simulink model "DK_Quydao_Control_PID1"  (R2020b)
settings: Solver=VariableStepAuto  StartTime=0.0  StopTime=20  RelTol=1e-3
undefined symbols (not defined in the file or in its folder): Kd1, Kd2, Ki1, Ki2, Kp1, Kp2
settings Model: Creator=ADMIN  LastModifiedBy=Admin
settings DataIOCC: ReturnWorkspaceOutputs=off
settings DebuggingCC: ArithmeticOperatorsInVariantConditions=warning
settings SFSimCC: CustomCodeUndefinedFunction=UseInterfaceOnly

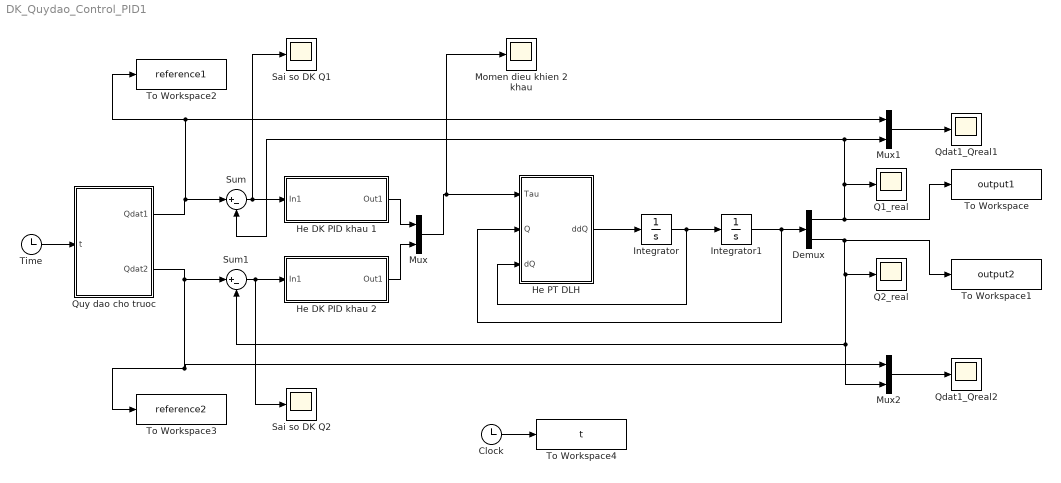
== system DK_Quydao_Control_PID1 ==
  Clock : Clock
  Demux : Demux  Outputs=2
  He DK PID khau 1 : Subsystem
  He DK PID khau 2 : Subsystem
  He PT DLH : MATLAB Function  TreatAsAtomicUnit=on
  Integrator : Integrator
  Integrator1 : Integrator  InitialCondition=[0;2]
  Momen dieu khien 2 khau : Scope
  Mux : Mux  Inputs=2
  Mux1 : Mux  Inputs=2
  Mux2 : Mux  Inputs=2
  Q1_real : Scope
  Q2_real : Scope
  Qdat1_Qreal1 : Scope
  Qdat1_Qreal2 : Scope
  Quy dao cho truoc : MATLAB Function  TreatAsAtomicUnit=on
  Sai so DK Q1 : Scope
  Sai so DK Q2 : Scope
  Sum : Sum  Inputs=|+-
  Sum1 : Sum  Inputs=|+-
  Time : Clock
  To Workspace : ToWorkspace  VariableName=output1  SampleTime=-1
  To Workspace1 : ToWorkspace  VariableName=output2  SampleTime=-1
  To Workspace2 : ToWorkspace  VariableName=reference1  SampleTime=-1
  To Workspace3 : ToWorkspace  VariableName=reference2  SampleTime=-1
  To Workspace4 : ToWorkspace  VariableName=t  SampleTime=-1
  wires:
  He PT DLH/1(ddQ) -> Integrator/1
  Mux/1 -> Momen dieu khien 2 khau/1, He PT DLH/1(Tau)
  He DK PID khau 1/1(Out1) -> Mux/1
  He DK PID khau 2/1(Out1) -> Mux/2
  Sum/1 -> Sai so DK Q1/1, He DK PID khau 1/1(In1)
  Quy dao cho truoc/1(Qdat1) -> Mux1/1, To Workspace2/1, Sum/1
  Sum1/1 -> Sai so DK Q2/1, He DK PID khau 2/1(In1)
  Quy dao cho truoc/2(Qdat2) -> Sum1/1, To Workspace3/1, Mux2/1
  Mux2/1 -> Qdat1_Qreal2/1
  Mux1/1 -> Qdat1_Qreal1/1
  Integrator1/1 -> He PT DLH/2(Q), Demux/1
  Integrator/1 -> He PT DLH/3(dQ), Integrator1/1
  Demux/1 -> To Workspace/1, Sum/2, Mux1/2, Q1_real/1
  Demux/2 -> To Workspace1/1, Sum1/2, Mux2/2, Q2_real/1
  Time/1 -> Quy dao cho truoc/1(t)
  Clock/1 -> To Workspace4/1

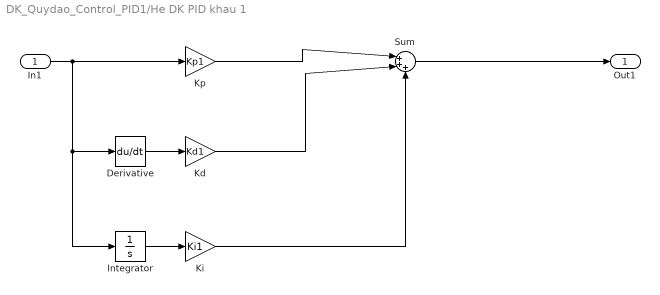
== system DK_Quydao_Control_PID1/He DK PID khau 1 ==
  In1 : Inport
  Derivative : Derivative
  Integrator : Integrator
  Kd : Gain  Gain=Kd1
  Ki : Gain  Gain=Ki1
  Kp : Gain  Gain=Kp1
  Sum : Sum  Inputs=|+++
  Out1 : Outport  VectorParamsAs1DForOutWhenUnconnected=off
  wires:
  In1/1 -> Derivative/1, Integrator/1, Kp/1
  Kp/1 -> Sum/1
  Integrator/1 -> Ki/1
  Derivative/1 -> Kd/1
  Kd/1 -> Sum/2
  Ki/1 -> Sum/3
  Sum/1 -> Out1/1

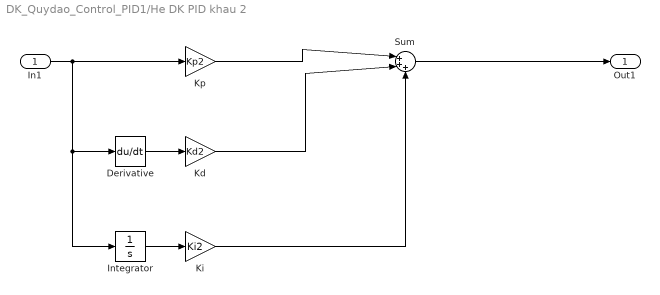
== system DK_Quydao_Control_PID1/He DK PID khau 2 ==
  In1 : Inport
  Derivative : Derivative
  Integrator : Integrator
  Kd : Gain  Gain=Kd2
  Ki : Gain  Gain=Ki2
  Kp : Gain  Gain=Kp2
  Sum : Sum  Inputs=|+++
  Out1 : Outport  VectorParamsAs1DForOutWhenUnconnected=off
  wires:
  Sum/1 -> Out1/1
  Ki/1 -> Sum/3
  Kd/1 -> Sum/2
  Derivative/1 -> Kd/1
  Integrator/1 -> Ki/1
  Kp/1 -> Sum/1
  In1/1 -> Kp/1, Integrator/1, Derivative/1

== matlab function DK_Quydao_Control_PID1/Quy dao cho truoc ==
  data: t input; Qdat1 output; Qdat2 output
function [Qdat1,Qdat2] = fcn(t)
Qdat1=0.5*sin(0.5*t);
Qdat2=1+cos(0.5*t);

== matlab function DK_Quydao_Control_PID1/He PT DLH ==
  data: Tau input; Q input; dQ input; ddQ output
function ddQ = fcn(Tau,Q,dQ)
[L1,Lc1,L2,Lc2,b,M1,M2,I1,I2,g]=parameter();
%%
ddQ=zeros(2,1);
%% Ma tran quan tinh (khoi luong suy rong)
Mq=zeros(2,2);
Mq(1,1)=M1*Lc1^2+M2*Lc2^2+M2*L1^2+2*M2*L1*Lc2*cos(Q(2))+I1+I2; 
Mq(1,2)=M2*Lc2^2+M2*L1*Lc2*cos(Q(2))+I2; 
Mq(2,1)=M2*Lc2^2+M2*L1*Lc2*cos(Q(2))+I2; 
Mq(2,2)=M2*Lc2^2+I2; 
%% Ma tran C
Cq=zeros(2,1);
Cq(1,1)=-2*M2*L1*Lc2*sin(Q(2))*dQ(1)*dQ(2)-M2*L1*Lc2*sin(Q(2))*dQ(2)^2; 
Cq(2,1)=M2*L1*Lc2*sin(Q(2))*dQ(1)^2; 
%% Ma tran trong truong
Gq=zeros(2,1);
Gq(1,1)=(M1*Lc1+M2*L1)*g*cos(Q(1))+M2*g*Lc2*cos(Q(1)+Q(2)); 
Gq(2,1)=M2*g*Lc2*cos(Q(1)+Q(2)); 
%% Phuong trinh dong luc hoc thuan
ddQ=inv(Mq)*(Tau-Cq-Gq);
